simulink model "ProposedProblem3"  (R2013a)
settings: Solver=ode45  StartTime=0.0  StopTime=14400  RelTol=1e-3
undefined symbols (not defined in the file): des, gcbh
settings Model: Creator=gabig  LastModifiedBy=gabig

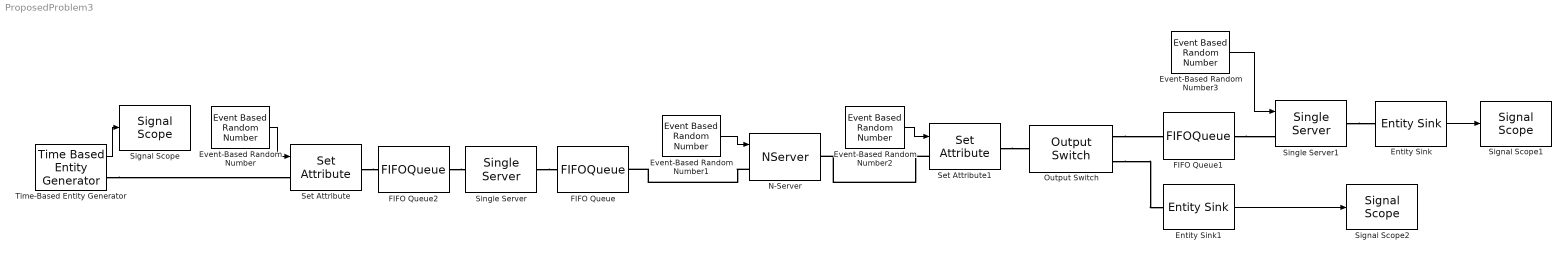
== system ProposedProblem3 ==
  Entity Sink : EntitySink  StatNumberArrived=on
  Entity Sink1 : EntitySink  StatNumberArrived=on
  Event-Based Random Number : EventBasedRandomNumber  Distribution=Uniform  minUnif=40  maxUnif=80  Seed=12360
  Event-Based Random Number1 : EventBasedRandomNumber  Distribution=Uniform  minUnif=120  maxUnif=240  valueVecDisc=[1 2]  probVecDisc=[0.3 0.7]  Seed=12337
  Event-Based Random Number2 : EventBasedRandomNumber  Distribution=Arbitrary discrete  valueVecDisc=[1 2]  probVecDisc=[0.3 0.7]  Seed=12331
  Event-Based Random Number3 : EventBasedRandomNumber  Distribution=Uniform  minUnif=70  maxUnif=170  Seed=12348
  FIFO Queue : FIFOQueue
  FIFO Queue1 : FIFOQueue
  FIFO Queue2 : FIFOQueue
  N-Server : NServer  NumberOfServers=1  ServiceTimeFrom=Signal port t
  Output Switch : OutputSwitch  NumberOutputPorts=2  SwitchingCriterion=From attribute  AttributeName=SERVICE
  Set Attribute : SetAttribute  AttributeName=LOADING  AttributeFrom=Signal port  EvaluatedAttributeValue={ []}
  Set Attribute1 : SetAttribute  AttributeName=SERVICE  AttributeFrom=Signal port  EvaluatedAttributeValue={ []}
  Signal Scope : SignalScope  LoadFcn=des.scope.CallbackSupport('seLoadFcn',gcbh)  StartFcn=des.scope.CallbackSupport('seStartFcn',gcbh)  StopFcn=des.scope.CallbackSupport('seStopFcn',gcbh)
      settings: CopyFcn=des.scope.CallbackSupport('seCopyFcn',gcbh)  DeleteFcn=des.scope.CallbackSupport('seDeleteFcn',gcbh)  PreSaveFcn=des.scope.CallbackSupport('sePreSaveFcn',gcbh)  NameChangeFcn=des.scope.CallbackSupport('seNameChangeFcn',gcbh)  OpenFcn=des.scope.CallbackSupport('seOpenFcn',gcbh)
  Signal Scope1 : SignalScope  LoadFcn=des.scope.CallbackSupport('seLoadFcn',gcbh)  StartFcn=des.scope.CallbackSupport('seStartFcn',gcbh)  StopFcn=des.scope.CallbackSupport('seStopFcn',gcbh)
      settings: CopyFcn=des.scope.CallbackSupport('seCopyFcn',gcbh)  DeleteFcn=des.scope.CallbackSupport('seDeleteFcn',gcbh)  PreSaveFcn=des.scope.CallbackSupport('sePreSaveFcn',gcbh)  NameChangeFcn=des.scope.CallbackSupport('seNameChangeFcn',gcbh)  OpenFcn=des.scope.CallbackSupport('seOpenFcn',gcbh)
  Signal Scope2 : SignalScope  LoadFcn=des.scope.CallbackSupport('seLoadFcn',gcbh)  StartFcn=des.scope.CallbackSupport('seStartFcn',gcbh)  StopFcn=des.scope.CallbackSupport('seStopFcn',gcbh)
      settings: CopyFcn=des.scope.CallbackSupport('seCopyFcn',gcbh)  DeleteFcn=des.scope.CallbackSupport('seDeleteFcn',gcbh)  PreSaveFcn=des.scope.CallbackSupport('sePreSaveFcn',gcbh)  NameChangeFcn=des.scope.CallbackSupport('seNameChangeFcn',gcbh)  OpenFcn=des.scope.CallbackSupport('seOpenFcn',gcbh)
  Single Server : SingleServer  ServiceTimeFrom=Attribute  AttributeName=LOADING
  Single Server1 : SingleServer  ServiceTimeFrom=Signal port t
  Time-Based Entity Generator : TimeBasedEntityGenerator  Distribution=Uniform  InitialSeed=12350  Minimum=60  Maximum=180  StatNumberDeparted=on
  wires:
  Event-Based Random Number/1 -> Set Attribute/1
  Event-Based Random Number2/1 -> Set Attribute1/1
  Time-Based Entity Generator/1 -> Signal Scope/1
  Entity Sink/1 -> Signal Scope1/1
  Entity Sink1/1 -> Signal Scope2/1
  Event-Based Random Number1/1 -> N-Server/1
  Event-Based Random Number3/1 -> Single Server1/1
  connections:
  Single Server1/RConn1 -- Entity Sink/LConn1
  Set Attribute1/LConn1 -- N-Server/RConn1
  Time-Based Entity Generator/RConn1 -- Set Attribute/LConn1
  Output Switch/RConn1 -- FIFO Queue1/LConn1
  N-Server/LConn1 -- FIFO Queue/RConn1
  Output Switch/RConn2 -- Entity Sink1/LConn1
  FIFO Queue1/RConn1 -- Single Server1/LConn1
  Set Attribute1/RConn1 -- Output Switch/LConn1
  FIFO Queue2/RConn1 -- Single Server/LConn1
  Set Attribute/RConn1 -- FIFO Queue2/LConn1
  Single Server/RConn1 -- FIFO Queue/LConn1
